simulink model "vehicle_model_skeleton"  (Simulink 7.0)
settings: Solver=ode45  StartTime=0.0  StopTime=10  MaxStep=0.01  RelTol=1e-3
settings Model: Creator=igo  LastModifiedBy=ibesseli
settings OptimizationCC: InitFltsAndDblsToZero=off
settings DebuggingCC: StrictBusMsg=ErrorLevel1

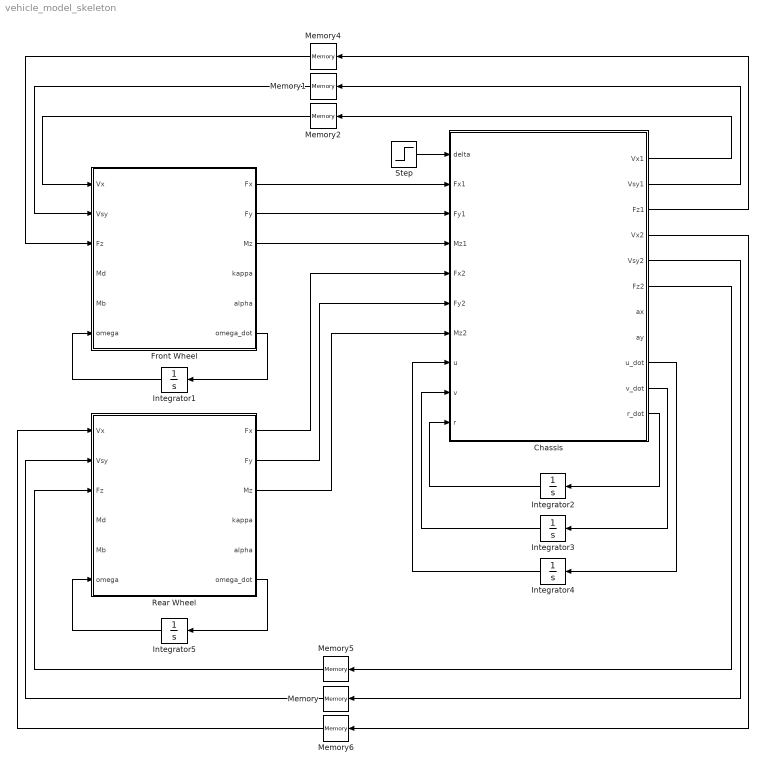
== system vehicle_model_skeleton ==
  Chassis : Stateflow chart
  Front Wheel : Stateflow chart  TreatAsAtomicUnit=on
  Integrator{1..5} (5 alike) : Integrator  Orientation=left
  Memory{,1..2,4..6} (6 alike) : Memory  Orientation=left
  Rear Wheel : Stateflow chart  TreatAsAtomicUnit=on
  Step : Step  After=0  SampleTime=0
  wires:
  Front Wheel/1(Fx) -> Chassis/2(Fx1)
  Step/1 -> Chassis/1(delta)
  Chassis/11(r_dot) -> Integrator2/1
  Integrator2/1 -> Chassis/10(r)
  Chassis/10(v_dot) -> Integrator3/1
  Integrator3/1 -> Chassis/9(v)
  Chassis/9(u_dot) -> Integrator4/1
  Integrator4/1 -> Chassis/8(u)
  Chassis/2(Vsy1) -> Memory1/1
  Chassis/5(Vsy2) -> Memory/1
  Chassis/1(Vx1) -> Memory2/1
  Memory2/1 -> Front Wheel/1(Vx)
  Memory1/1 -> Front Wheel/2(Vsy)
  Chassis/3(Fz1) -> Memory4/1
  Memory4/1 -> Front Wheel/3(Fz)
  Rear Wheel/1(Fx) -> Chassis/5(Fx2)
  Rear Wheel/2(Fy) -> Chassis/6(Fy2)
  Memory/1 -> Rear Wheel/2(Vsy)
  Chassis/4(Vx2) -> Memory6/1
  Memory6/1 -> Rear Wheel/1(Vx)
  Memory5/1 -> Rear Wheel/3(Fz)
  Chassis/6(Fz2) -> Memory5/1
  Front Wheel/6(omega_dot) -> Integrator1/1
  Integrator1/1 -> Front Wheel/6(omega)
  Rear Wheel/6(omega_dot) -> Integrator5/1
  Integrator5/1 -> Rear Wheel/6(omega)
  Front Wheel/2(Fy) -> Chassis/3(Fy1)
  Front Wheel/3(Mz) -> Chassis/4(Mz1)
  Rear Wheel/3(Mz) -> Chassis/7(Mz2)

== matlab function Front Wheel ==
  data: Vx input double; Fx output double; Vsy input double; Fz input double; Md input double; Mb input inherited; Fy output double; Mz output double; kappa output double; alpha output double; omega input inherited; omega_dot output inherited
function [Fx,Fy,Mz,kappa,alpha,omega_dot]=brush_tyre(Vx,Vsy,Fz,Md,Mb,omega)

Fx=0;
Fy=0;
Mz=0;
kappa=0;
alpha=0;
omega_dot=0;

return

== matlab function Rear Wheel ==
  data: Vx input double; Fx output double; Vsy input double; Fz input double; Md input double; Mb input inherited; Fy output double; Mz output double; kappa output double; alpha output double; omega input inherited; omega_dot output inherited
function [Fx,Fy,Mz,kappa,alpha,omega_dot]=brush_tyre(Vx,Vsy,Fz,Md,Mb,omega)

Fx=0;
Fy=0;
Mz=0;
kappa=0;
alpha=0;
omega_dot=0;

return

== matlab function Chassis ==
  data: delta input inherited; Fx1 input inherited; Fy1 input inherited; Mz1 input inherited; Fx2 input inherited; Fy2 input inherited; Mz2 input inherited; u input inherited; Vx1 output inherited; v input inherited; r input inherited; Vsy1 output inherited; Fz1 output inherited; Vx2 output inherited; Vsy2 output inherited; Fz2 output inherited; ax output inherited; ay output inherited; u_dot output inherited; v_dot output inherited; r_dot output inherited
function [Vx1,Vsy1,Fz1,Vx2,Vsy2,Fz2,ax,ay,u_dot,v_dot,r_dot] = chassis_dynamics(delta,Fx1,Fy1,Mz1,Fx2,Fy2,Mz2,u,v,r)

Vx1=0;
Vsy1=0;
Fz1=0;
Vx2=0;
Vsy2=0;
Fz2=0;
ax=0;
ay=0;
u_dot=0;
v_dot=0;
r_dot=0;

return
